simulink model "blockdemo"  (Simulink 6.3)
settings: Solver=FixedStepDiscrete  StartTime=0.0  StopTime=50  RelTol=1e-3
InitFcn:
  | %% DSPBuilder Start
  | alt_dspbuilder_update_model(bdroot)
  | %% DSPBuilder End
libraries: allblocks_alteradspbuilder2 x4
settings Model: LastModifiedBy=delphick

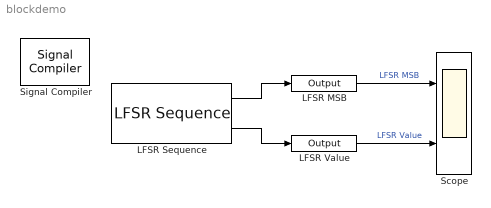
== system blockdemo ==
  LFSR MSB : allblocks_alteradspbuilder2/Output  iofile=C:\workspace_clean\Documentation\DesignExamples\Tutorials\UnitBlocks\GateAndControl\LFSRSequence\tb_blockdemo\blockdemo_LFSR+MSB.capture  BusType=Single Bit  bwl=8  bwr=0  PORTTYPE=Output
  LFSR Sequence : allblocks_alteradspbuilder2/LFSR Sequence  length=10  feedback_structure=External n-inputs gate (many-to-one)  feedback_gate_type=XOR  initial_reg_val_hex=FFFFFFFF  initial_reg_val_bin=1111111111  poly_tap_seq=[0 3 10]  poly_tap_seq_bin=1000000100  SpecifyClock=off  use_parallel_out=on  use_ena=off  use_sclr=off
  LFSR Value : allblocks_alteradspbuilder2/Output  iofile=C:\workspace_clean\Documentation\DesignExamples\Tutorials\UnitBlocks\GateAndControl\LFSRSequence\tb_blockdemo\blockdemo_LFSR+Value.capture  BusType=Unsigned Integer  bwl=10  bwr=0  PORTTYPE=Output
  Scope : Scope  NumInputPorts=2
      settings: TimeRange=50  YMin=-2~0  YMax=2~1200
  Signal Compiler : allblocks_alteradspbuilder2/Signal Compiler  DeviceFamily=Stratix IV  DeviceName=AUTO  EnableSignalTap=off  SignalTapDepth=128  UseBoardBlock=off  StpUseDefaultClock=on  StpClock=clock
  wires:
  LFSR Sequence/1 -> LFSR MSB/1
  LFSR Sequence/2 -> LFSR Value/1
  LFSR MSB/1 -> Scope/1  "LFSR MSB"
  LFSR Value/1 -> Scope/2  "LFSR Value"
